simulink model "Example6a"  (Simulink 6.0)
settings: Solver=ode45  StartTime=0.0  StopTime=10.0  RelTol=1e-3
settings Model: LastModifiedBy=Administrator

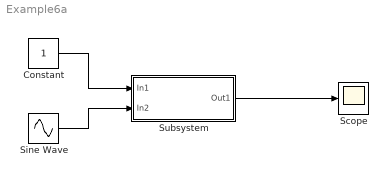
== system Example6a ==
  Constant : Constant
  Scope : Scope
  Sine Wave : Sin  SampleTime=0
  Subsystem : Subsystem
  wires:
  Constant/1 -> Subsystem/1(In1)
  Sine Wave/1 -> Subsystem/2(In2)
  Subsystem/1(Out1) -> Scope/1

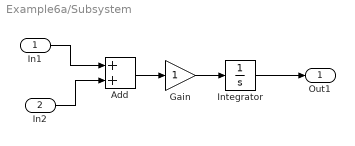
== system Example6a/Subsystem ==
  In1 : Inport  Port=1  LatchInput=off
  In2 : Inport  Port=2  LatchInput=off
  Add : Sum  OutScaling=2^-10
  Gain : Gain
  Integrator : Integrator
  Out1 : Outport
  wires:
  In1/1 -> Add/1
  In2/1 -> Add/2
  Add/1 -> Gain/1
  Gain/1 -> Integrator/1
  Integrator/1 -> Out1/1
